simulink model "BPSK_carr_rec"  (R2023b)
settings: Solver=ode45  StartTime=0.0  StopTime=20  MaxStep=0.01  MinStep=0.001  RelTol=1e-3  EnableMultiTasking=on
libraries: dspfdesign x2, simulink_extras x1, simulink x1
settings Model: Creator=SIMONA  LastModifiedBy=adiicmp_
settings SolverCC: AlgebraicLoopSolver=TrustRegion
settings DataIOCC: LimitDataPoints=on  SaveFormat=Array  ReturnWorkspaceOutputs=off
settings OptimizationCC: LifeSpan=inf
settings DebuggingCC: UnconnectedInputMsg=warning  UnconnectedOutputMsg=warning  UnconnectedLineMsg=warning  SFUnexpectedBacktrackingDiag=warning  SFNoUnconditionalDefaultTransitionDiag=warning  ArithmeticOperatorsInVariantConditions=warning
settings HardwareCC: ProdBitPerPointer=32  ProdBitPerSizeT=32  ProdBitPerPtrDiffT=32  ProdLargestAtomicFloat=None  ProdIntDivRoundTo=Undefined  ProdEndianess=Unspecified  ProdWordSize=32  ProdHWDeviceType=32-bit Generic
settings ModelReferenceCC: EnableRefExpFcnMdlSchedulingChecks=on  PropagateSignalLabelsOutOfModel=off
settings SFSimCC: SimUseLocalCustomCode=off  CustomCodeUndefinedFunction=UseInterfaceOnly
settings RTWCC: RTWUseLocalCustomCode=off
settings CodeAppCC: StateflowObjectComments=on
settings GRTTargetCC: TargetLangStandard=C89/C90 (ANSI)
settings ConfigComp: CovMetricSettings=dw  CovSaveCumulativeToWorkspaceVar=on  CovSaveSingleToWorkspaceVar=on  CovExternalEMLEnable=off

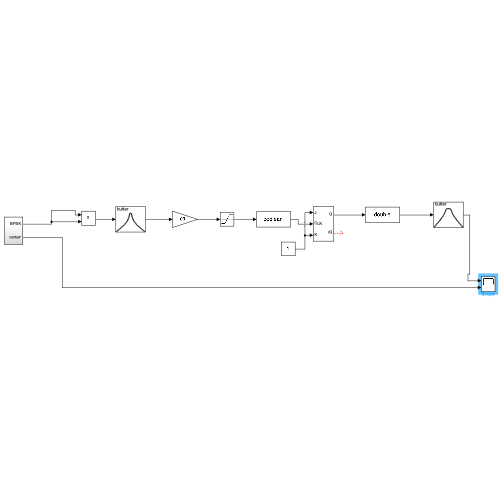
[thumbnail: Simulink's stored preview of the top-level diagram]
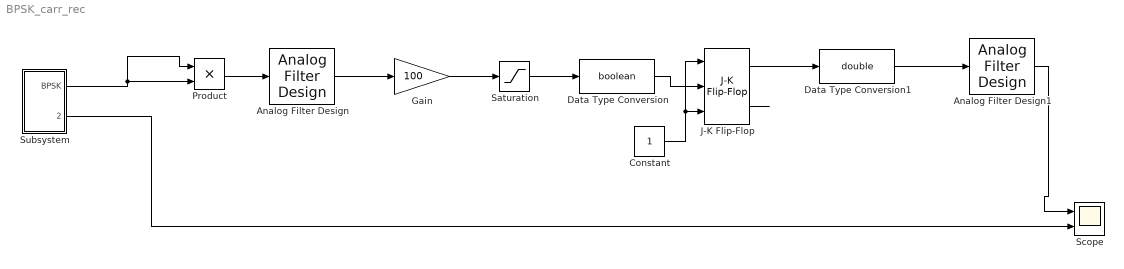
== system BPSK_carr_rec ==
  Analog Filter Design : dspfdesign/Analog Filter Design  method=Butterworth  filttype=Bandpass  N=10  Wlo=2*pi*2*10*(1-0.1)  Whi=2*pi*2*10*(1+0.1)  Rp=2  Rs=40
  Analog Filter Design1 : dspfdesign/Analog Filter Design  method=Butterworth  filttype=Bandpass  N=10  Wlo=pi*2*10*0.7  Whi=pi*2*10*1.3  Rp=2  Rs=40
  Constant : Constant  OutDataTypeStr=boolean
  Data Type Conversion : DataTypeConversion  OutDataTypeStr=boolean  SaturateOnIntegerOverflow=off  RndMeth=Floor
  Data Type Conversion1 : DataTypeConversion  OutDataTypeStr=double  SaturateOnIntegerOverflow=off  RndMeth=Floor
  Gain : Gain  Gain=100
  J-K Flip-Flop : simulink_extras/Flip Flops/J-K Flip-Flop  initial_condition=0
  Product : Product
  Saturation : Saturate  UpperLimit=1  LowerLimit=0
  Scope : Scope  NumInputPorts=2
  Subsystem : Subsystem
  wires:
  Subsystem/2(carrier) -> Scope/2
  Gain/1 -> Saturation/1
  Analog Filter Design/1 -> Gain/1
  Saturation/1 -> Data Type Conversion/1
  Subsystem/1(BPSK) -> Product/1, Product/2
  Product/1 -> Analog Filter Design/1
  Data Type Conversion/1 -> J-K Flip-Flop/2
  Analog Filter Design1/1 -> Scope/1
  Data Type Conversion1/1 -> Analog Filter Design1/1
  Constant/1 -> J-K Flip-Flop/1, J-K Flip-Flop/3
  J-K Flip-Flop/1 -> Data Type Conversion1/1
  J-K Flip-Flop/2 -> ?

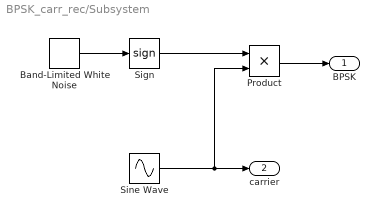
== system BPSK_carr_rec/Subsystem ==
  Band-Limited White Noise : simulink/Sources/Band-Limited White Noise  Cov=[0.1]  Ts=1  seed=[23341]
  Product : Product
  Sign : Signum
  Sine Wave : Sin  Bias=4  Frequency=2*pi*10  SampleTime=0
  BPSK : Outport
  carrier : Outport  Port=2
  wires:
  Product/1 -> BPSK/1
  Sine Wave/1 -> Product/2, carrier/1
  Band-Limited White Noise/1 -> Sign/1
  Sign/1 -> Product/1
